simulink library "Lib_Solve_OuterLoopIntegrator_TMATS_org"  (Simulink 10.0)
settings: Solver=ode45  StartTime=0.0  StopTime=10.0  RelTol=1e-3  EnableMultiTasking=on
Description:
  | Thomas Modules
settings Model: Creator=jwchapm2  LastModifiedBy=bhisma

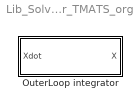
== system Lib_Solve_OuterLoopIntegrator_TMATS_org ==
  OuterLoop integrator : Subsystem  mask(T-MATS: OuterLoop Integrator Library Block){OL_IC_M=10000}
      mask prompts: OL_IC_M "OL_IC_M - Model Outer Loop Initial Conditions"
      mask help: Continuous-time integration of the input signal. To be used in the simulations outer, time based, loop.
      mask Help: web(which('Solver_TMATS_OLI.html'),'-helpbrowser')

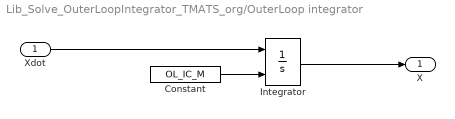
== system Lib_Solve_OuterLoopIntegrator_TMATS_org/OuterLoop integrator ==
  Xdot : Inport
  Constant : Constant  Value=OL_IC_M
  Integrator : Integrator  InitialConditionSource=external
  X : Outport
  wires:
  Constant/1 -> Integrator/2
  Xdot/1 -> Integrator/1
  Integrator/1 -> X/1
